simulink model "simulink_tasks"  (R2024a)
settings: Solver=VariableStepAuto  StartTime=0.0  StopTime=10.0  RelTol=1e-3
libraries: cstblocks x12, simulink x12
settings Model: Creator=SHAHZAD BANGASH  LastModifiedBy=SHAHZAD BANGASH

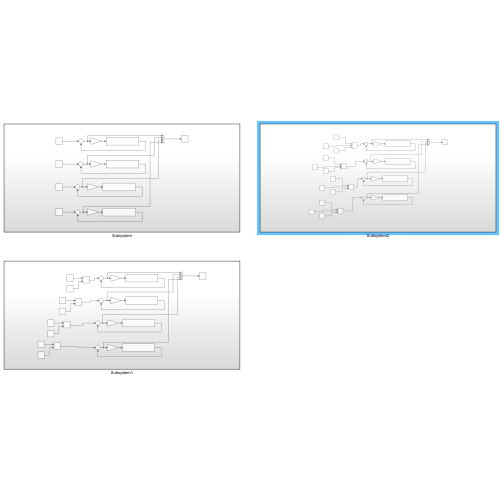
[thumbnail: Simulink's stored preview of the top-level diagram]
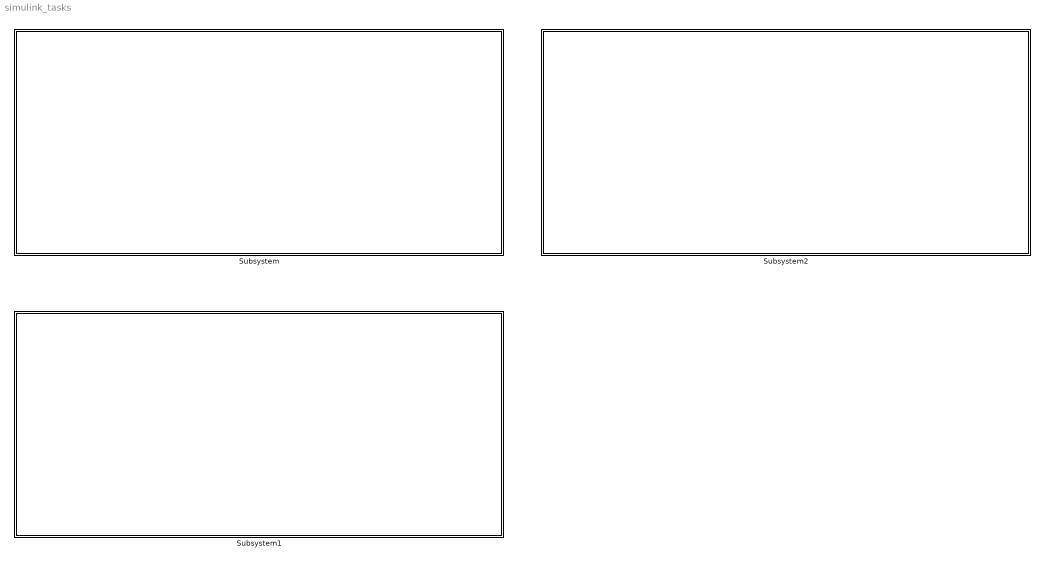
== system simulink_tasks ==
  Subsystem : Subsystem
  Subsystem1 : Subsystem
  Subsystem2 : Subsystem

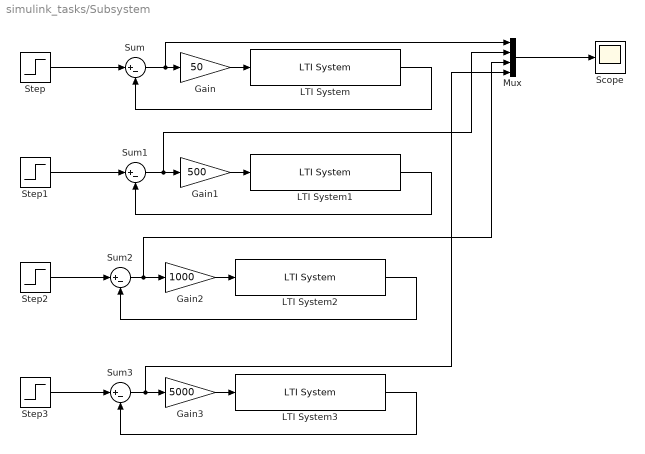
== system simulink_tasks/Subsystem ==
  Gain : Gain  Gain=50
  Gain1 : Gain  Gain=500
  Gain2 : Gain  Gain=1000
  Gain3 : Gain  Gain=5000
  LTI System{,1..3} (4 alike) : cstblocks/LTI System  sys=tf([1 6], [1, 32, 367, 1776 , 3024])  IC=[]  PadeOrder=0
  Mux : Mux
  Scope : Scope
  Step{,1..3} (4 alike) : Step  Time=0  After=5  SampleTime=0
  Sum{,1..3} (4 alike) : Sum  Inputs=|+-
  wires:
  Step/1 -> Sum/1
  Sum/1 -> Mux/1, Gain/1
  Gain/1 -> LTI System/1
  Gain1/1 -> LTI System1/1
  LTI System3/1 -> Sum3/2
  Step1/1 -> Sum1/1
  LTI System/1 -> Sum/2
  Sum1/1 -> Mux/2, Gain1/1
  LTI System1/1 -> Sum1/2
  Sum3/1 -> Mux/4, Gain3/1
  Gain3/1 -> LTI System3/1
  Step3/1 -> Sum3/1
  Mux/1 -> Scope/1
  Sum2/1 -> Mux/3, Gain2/1
  Step2/1 -> Sum2/1
  Gain2/1 -> LTI System2/1
  LTI System2/1 -> Sum2/2

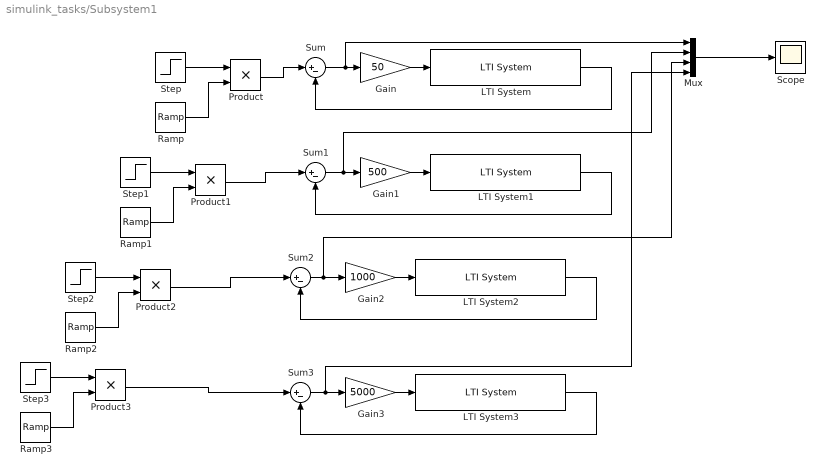
== system simulink_tasks/Subsystem1 ==
  Gain : Gain  Gain=50
  Gain1 : Gain  Gain=500
  Gain2 : Gain  Gain=1000
  Gain3 : Gain  Gain=5000
  LTI System{,1..3} (4 alike) : cstblocks/LTI System  sys=tf([1 6], [1, 32, 367, 1776 , 3024])  IC=[]  PadeOrder=0
  Mux : Mux
  Product{,1..3} (4 alike) : Product
  Ramp{,1..3} (4 alike) : simulink/Sources/Ramp  slope=1  start=0  InitialOutput=0
  Scope : Scope
  Step{,1..3} (4 alike) : Step  Time=0  After=5  SampleTime=0
  Sum{,1..3} (4 alike) : Sum  Inputs=|+-
  wires:
  Sum/1 -> Mux/1, Gain/1
  Gain/1 -> LTI System/1
  Gain1/1 -> LTI System1/1
  LTI System3/1 -> Sum3/2
  LTI System/1 -> Sum/2
  Sum1/1 -> Mux/2, Gain1/1
  LTI System1/1 -> Sum1/2
  Sum3/1 -> Mux/4, Gain3/1
  Gain3/1 -> LTI System3/1
  Mux/1 -> Scope/1
  Sum2/1 -> Mux/3, Gain2/1
  Gain2/1 -> LTI System2/1
  LTI System2/1 -> Sum2/2
  Step/1 -> Product/1
  Ramp/1 -> Product/2
  Product/1 -> Sum/1
  Product1/1 -> Sum1/1
  Ramp1/1 -> Product1/2
  Step1/1 -> Product1/1
  Product2/1 -> Sum2/1
  Ramp2/1 -> Product2/2
  Step2/1 -> Product2/1
  Product3/1 -> Sum3/1
  Ramp3/1 -> Product3/2
  Step3/1 -> Product3/1

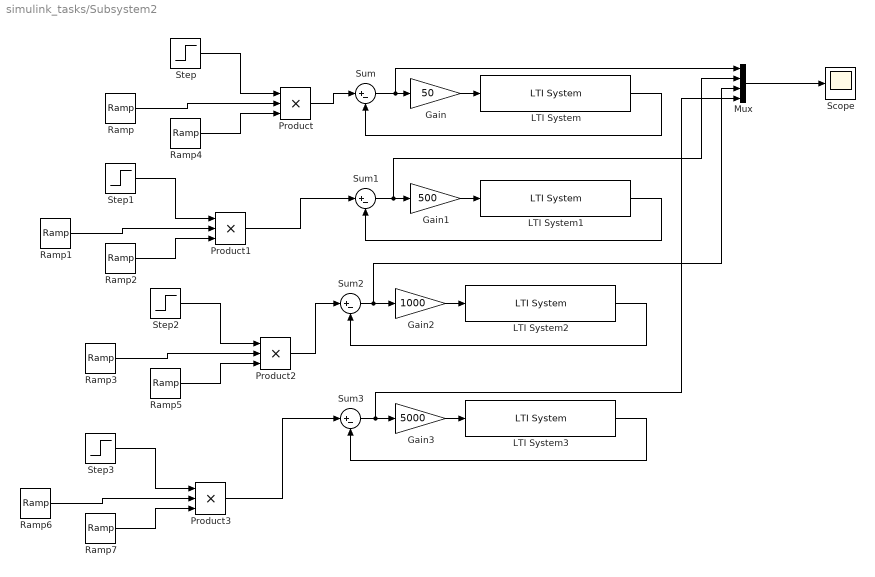
== system simulink_tasks/Subsystem2 ==
  Gain : Gain  Gain=50
  Gain1 : Gain  Gain=500
  Gain2 : Gain  Gain=1000
  Gain3 : Gain  Gain=5000
  LTI System{,1..3} (4 alike) : cstblocks/LTI System  sys=tf([1 6], [1, 32, 367, 1776 , 3024])  IC=[]  PadeOrder=0
  Mux : Mux
  Product{,1..3} (4 alike) : Product  Inputs=3
  Ramp{,1..7} (8 alike) : simulink/Sources/Ramp  slope=1  start=0  InitialOutput=0
  Scope : Scope
  Step{,1..3} (4 alike) : Step  Time=0  After=5  SampleTime=0
  Sum{,1..3} (4 alike) : Sum  Inputs=|+-
  wires:
  Sum/1 -> Mux/1, Gain/1
  Gain/1 -> LTI System/1
  Gain1/1 -> LTI System1/1
  LTI System3/1 -> Sum3/2
  LTI System/1 -> Sum/2
  Sum1/1 -> Mux/2, Gain1/1
  LTI System1/1 -> Sum1/2
  Sum3/1 -> Mux/4, Gain3/1
  Gain3/1 -> LTI System3/1
  Mux/1 -> Scope/1
  Sum2/1 -> Mux/3, Gain2/1
  Gain2/1 -> LTI System2/1
  LTI System2/1 -> Sum2/2
  Step/1 -> Product/1
  Product/1 -> Sum/1
  Ramp/1 -> Product/2
  Ramp4/1 -> Product/3
  Ramp2/1 -> Product1/3
  Step1/1 -> Product1/1
  Ramp1/1 -> Product1/2
  Product1/1 -> Sum1/1
  Ramp5/1 -> Product2/3
  Step2/1 -> Product2/1
  Ramp3/1 -> Product2/2
  Product2/1 -> Sum2/1
  Ramp7/1 -> Product3/3
  Step3/1 -> Product3/1
  Ramp6/1 -> Product3/2
  Product3/1 -> Sum3/1
